simulink model "dmccontrol"  (R2014b)
settings: Solver=VariableStepAuto  StartTime=0.0  StopTime=Tstop  FixedStep=Ts  RelTol=1e-3
InitFcn:
  | dmc=dmcinit(Su,Sd,c,lambda,alfa,futref,r);
  | assignin('base','dmc',dmc);
values from neighbouring files (symbols this model uses):
  alfa = 1    [DMCejemplo.m]
  c = 1    [DMCejemplo.m]
  futref = 0')    [DMCejemplo.m]
  inputnoisegain = 0    [DMCejemplo.m]
  lambda = 1(r),50(k),100(m)    [DMCejemplo.m]
  outputnoisegain = 0    [DMCejemplo.m]
  r = [zeros(15/Ts,1); 12*ones(45/Ts,1)]    [DMCejemplo.m]
  steptimeDV = 35    [DMCejemplo.m]
  steptimeUDV = 45    [DMCejemplo.m]
  Ts = 0.5    [DMCejemplo.m]
  valueDV = 2    [DMCejemplo.m]
  valueUDV = -2    [DMCejemplo.m]
undefined symbols (not defined in the file): gdv, gu, gudv
libraries: cstblocks x3
settings Model: Creator=juaherdu  LastModifiedBy=juaherdu
settings DataIOCC: SaveFormat=Dataset
settings OptimizationCC: UseDivisionForNetSlopeComputation=off  SimCompilerOptimization=off
settings DebuggingCC: SolverPrmCheckMsg=none  FrameProcessingCompatibilityMsg=error  AllowSymbolicDim=off
settings HardwareCC: ProdBitPerPointer=64  ProdLargestAtomicFloat=Float  ProdIntDivRoundTo=Zero  ProdEndianess=LittleEndian  ProdWordSize=64  ProdHWDeviceType=Intel->x86-64 (Windows64)
settings RTWCC: RTWCompilerOptimization=off
settings GRTTargetCC: GeneratePreprocessorConditionals=Use local settings
settings ConfigComp: CovMetricSettings=dw  CovHtmlReporting=on  CovSaveCumulativeToWorkspaceVar=on  CovSaveSingleToWorkspaceVar=on  CovExternalEMLEnable=off

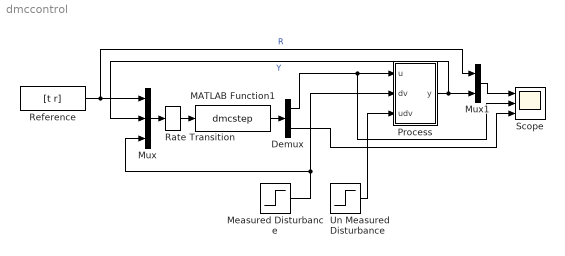
== system dmccontrol ==
  Demux : Demux  Outputs=2
  MATLAB Function1 : MATLABFcn  MATLABFcn=dmcstep  OutputDimensions=2  SampleTime=Ts
  Measured Disturbance : Step  Time=steptimeDV  After=valueDV  SampleTime=Ts
  Mux : Mux  Inputs=3
  Mux1 : Mux  Inputs=2
  Process : Subsystem  mask{gu=gu, gdv=gdv, gudv=gudv, inputnoisegain=inputnoisegain, outputnoisegain=outputnoisegain}
      mask prompts: gu "fdt y/u"; gdv "fdt y/dv"; gudv "fdt y/udv"; inputnoisegain "inputnoise"; outputnoisegain "outputnoise"
      mask DialogControl DescTextVar Prompt: Parametros del Modelo del proceso
  Rate Transition : RateTransition  OutPortSampleTime=Ts
  Reference : FromWorkspace  VariableName=[t r]  SampleTime=Ts
  Scope : Scope  NumInputPorts=3
      settings: ShowLegends=on  YMin=-1.65042~-1.65125~-0.54786  YMax=14.8538~14.86128~1.41344  SaveName=Simul  MaxDataPoints=50000
  Un Measured Disturbance : Step  Time=steptimeUDV  After=valueUDV  SampleTime=Ts
  wires:
  Measured Disturbance/1 -> Process/2(dv), Mux/3
  Un Measured Disturbance/1 -> Process/3(udv)
  Reference/1 -> Mux/1, Mux1/1  "R"
  Mux/1 -> Rate Transition/1
  Demux/1 -> Scope/2, Process/1(u)
  Process/1(y) -> Mux/2, Mux1/2  "Y"
  Mux1/1 -> Scope/1
  Demux/2 -> Scope/3
  Rate Transition/1 -> MATLAB Function1/1
  MATLAB Function1/1 -> Demux/1

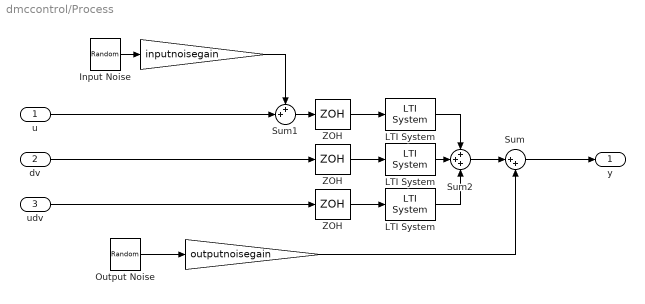
== system dmccontrol/Process ==
  u : Inport
  dv : Inport  Port=2
  udv : Inport  Port=3
  " " : Gain  Gain=inputnoisegain
  "  " : Gain  Gain=outputnoisegain
  " ZOH" : ZeroOrderHold  SampleTime=Ts
  Input Noise : UniformRandomNumber  SampleTime=Ts
  LTI System : cstblocks/LTI System  sys=gu  IC=[]
  "LTI System " : cstblocks/LTI System  sys=gdv  IC=[]
  "LTI System  " : cstblocks/LTI System  sys=gudv  IC=[]
  Output Noise : UniformRandomNumber  SampleTime=Ts
  Sum : Sum  Inputs=|++
  Sum1 : Sum  Inputs=++|
  Sum2 : Sum  Inputs=+++
  ZOH : ZeroOrderHold  SampleTime=Ts
  "ZOH " : ZeroOrderHold  SampleTime=Ts
  y : Outport
  wires:
  Sum/1 -> y/1
  dv/1 -> "ZOH "/1
  "  "/1 -> Sum/2
  udv/1 -> ZOH/1
  u/1 -> Sum1/2
  Sum2/1 -> Sum/1
  Output Noise/1 -> "  "/1
  Input Noise/1 -> " "/1
  Sum1/1 -> " ZOH"/1
  "LTI System  "/1 -> Sum2/3
  LTI System/1 -> Sum2/1
  "LTI System "/1 -> Sum2/2
  " "/1 -> Sum1/1
  " ZOH"/1 -> LTI System/1
  "ZOH "/1 -> "LTI System "/1
  ZOH/1 -> "LTI System  "/1
